simulink model "sprimd"  (Simulink 8.1)
settings: Solver=ode4  StartTime=0.0  StopTime=5.0  FixedStep=0.001  RelTol=1e-3
values from neighbouring files (symbols this model uses):
  k1 = 6000    [1.mat]    (also in 2.mat = 55000; 3.mat = 55000)
  m1 = 14000    [1.mat]    (also in 2.mat; 3.mat)
  v0 = 70    [1.mat]    (also in 2.mat; 3.mat = 67)
settings Model: Creator=student  LastModifiedBy=adasdeb
settings DataIOCC: TimeSaveName=tout_wpr_spr
settings DebuggingCC: FcnCallInpInsideContextMsg=EnableAllAsWarning
settings GRTTargetCC: CombineOutputUpdateFcns=on  GRTInterface=off

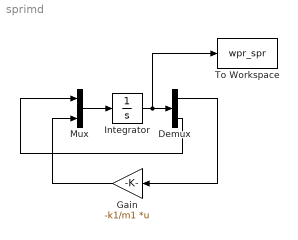
== system sprimd ==
  Demux : Demux  Outputs=2
  Gain : Gain  Gain=-k1/m1  Multiplication=Matrix(K*u)
  Integrator : Integrator  InitialCondition=[0;v0]
  Mux : Mux  Inputs=2
  To Workspace : ToWorkspace  VariableName=wpr_spr  SampleTime=-1  SaveFormat=Timeseries
  wires:
  Mux/1 -> Integrator/1
  Integrator/1 -> To Workspace/1, Demux/1
  Demux/1 -> Gain/1
  Gain/1 -> Mux/2
  Demux/2 -> Mux/1
